simulink model "quadrotorsim"  (Simulink 9.2)
settings: Solver=ode45  StartTime=0.0  StopTime=200  FixedStep=1  RelTol=1e-3  EnableMultiTasking=on
undefined symbols (not defined in the file): delta_th_lim, delta_w_lim, Fmat, Hmat, KfupdatePeriodInCycle, max_bias, Q, q0, qest0, R, Tcapt, TkfProp, Tqint
libraries: simulink x2
settings Model: Creator=samirbo  LastModifiedBy=william
settings OptimizationCC: ExpressionDepthLimit=2147483647  InitFltsAndDblsToZero=on
settings DebuggingCC: SaveWithParameterizedLinksMsg=none  SignalResolutionControl=TryResolveAllWithWarning  SolverPrmCheckMsg=warning  MultiTaskDSMMsg=warning  MultiTaskCondExecSysMsg=none
settings GRTTargetCC: TargetFcnLib=ansi_tfl_tmw.mat

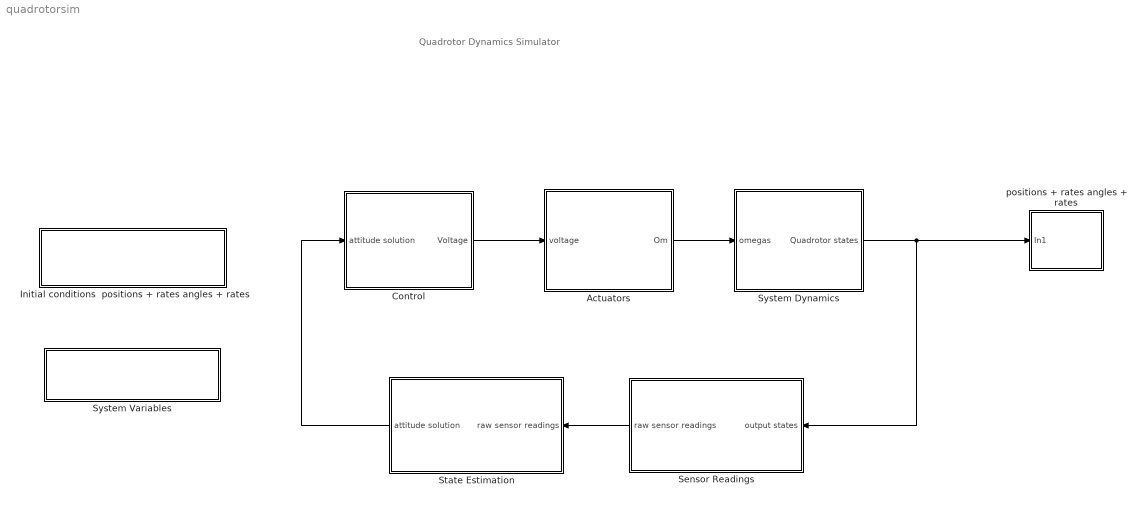
== system quadrotorsim ==
  note: Quadrotor Dynamics Simulator
  Actuators : Subsystem
      mask Display: image(imread('Brushless-motor.jpg'))
  Control : Subsystem
      mask Display: image(imread('control.bmp'))
  Initial conditions  positions + rates angles + rates : Subsystem  mask{x0=5, y0=5, z0=5, x0dot=1, y0dot=1, z0dot=1, phi0=0, theta0=0, psi0=0, phi0dot=0, theta0dot=0, psi0dot=0}
      mask prompts: x0 "Initial X position, in meters"; y0 "Initial Y position, in meters"; z0 "Initial Z position, in meters"; x0dot "Initial Velocity in X direction, m/sec"; y0dot "Initial Velocity in Y direction, m/sec"; z0dot "Initial Velocity in Z direction, m/sec"; phi0 "Initial Roll angle, deg"; theta0 "Initial Pitch angle, deg"; psi0 "Initial Yaw angle, deg"; phi0dot "Initial Roll rate, deg/sec"; theta0dot "Initial Pitch rate, deg/sec"; psi0dot "Initial Yaw rate, deg/sec"
      mask Display: disp('Enter initial conditions here')
  Sensor Readings : Subsystem
      mask Display: image(imread('imu.jpg'))
  State Estimation : Subsystem
      mask Display: image(imread('filter.png'))
  System Dynamics : Subsystem
      mask Display: image(imread('Quadrotor.png'))
  System Variables : Subsystem  mask{m=5, Ixx=0.03, Iyy=0.03, Izz=0.03, b=1, d=0.6, Jr=0.01, l=0.5}
      mask prompts: m "Quadrotor Mass, in kg"; Ixx "Quadrotor Moment of Inertia along x axis, in kg.m^2"; Iyy "Quadrotor Moment of Inertia along y axis, in kg.m^2"; Izz "Quadrotor Moment of Inertia along z axix, kg.m^2"; b "Thrust Factor"; d "Drag factor"; Jr "Rotor Inertia, in kg.m^2"; l "Length from the rotor to the centre of mass, in m"
      mask Display: disp('input system variables')
  positions + rates angles + rates : Subsystem
      mask Display: disp('system states')
  wires:
  Actuators/1(Om) -> System Dynamics/1(omegas)
  System Dynamics/1(Quadrotor states) -> Sensor Readings/1(output states), positions + rates angles + rates/1(In1)
  Sensor Readings/1(raw sensor readings) -> State Estimation/1(raw sensor readings)
  Control/1(Voltage) -> Actuators/1(voltage)
  State Estimation/1(attitude solution) -> Control/1(attitude solution)

== system quadrotorsim/Actuators ==
  voltage : Inport
  Bus Creator : BusCreator  Inputs=4
  Bus Selector : BusSelector  OutputSignals=d
  "Motor Dynamics - Front Motor " : Subsystem  mask{Jm=0.001, Jp=0.01, R=0.1, Ke=23}
      mask prompts: Jm "Total Moment of Inertia of the motor in the spin axis, N m s^2"; Jp "Total Moment of Inertia of the propeller in the spin axis, N m s^2"; R "Internal resistance of the motor, Ohm"; Ke "Motor constant, V/rad/sec"
  Motor Dynamics - Left Motor : Subsystem  mask{Jm=0.001, Jp=0.01, R=0.1, Ke=23}
      mask prompts: Jm "Total Moment of Inertia of the motor in the spin axis, N m s^2"; Jp "Total Moment of Inertia of the propeller in the spin axis, N m s^2"; R "Internal resistance of the motor, Ohm"; Ke "Motor constant, V/rad/sec"
  Motor Dynamics - Rear Motor : Subsystem  mask{Jm=0.001, Jp=0.01, R=0.1, Ke=23}
      mask prompts: Jm "Total Moment of Inertia of the motor in the spin axis, N m s^2"; Jp "Total Moment of Inertia of the propeller in the spin axis, N m s^2"; R "Internal resistance of the motor, Ohm"; Ke "Motor constant, V/rad/sec"
  Motor Dynamics - Right Motor : Subsystem  mask{Jm=0.001, Jp=0.01, R=0.1, Ke=23}
      mask prompts: Jm "Total Moment of Inertia of the motor in the spin axis, N m s^2"; Jp "Total Moment of Inertia of the propeller in the spin axis, N m s^2"; R "Internal resistance of the motor, Ohm"; Ke "Motor constant, V/rad/sec"
  Om : Outport
  wires:
  [SystemVariables] -> Bus Selector/1
  Bus Selector/1 -> Motor Dynamics - Right Motor/2(drag coefficient), Motor Dynamics - Rear Motor/2(drag coefficient), Motor Dynamics - Left Motor/2(drag coefficient), "Motor Dynamics - Front Motor "/2(drag coefficient)  "<d>"
  voltage/1 -> "Motor Dynamics - Front Motor "/1(voltage), Motor Dynamics - Right Motor/1(voltage), Motor Dynamics - Rear Motor/1(voltage), Motor Dynamics - Left Motor/1(voltage)
  "Motor Dynamics - Front Motor "/1(RPS) -> Bus Creator/1  "Om_1"
  Motor Dynamics - Right Motor/1(RPS) -> Bus Creator/2  "Om_2"
  Motor Dynamics - Rear Motor/1(RPS) -> Bus Creator/3  "Om_3"
  Motor Dynamics - Left Motor/1(RPS) -> Bus Creator/4  "Om_4"
  Bus Creator/1 -> Om/1

== system quadrotorsim/Control ==
  attitude solution : Inport
  Bus Selector : BusSelector  OutputSignals=west
  Voltage conversion : Gain
  attitude controller : Subsystem
  steering commands : Subsystem
  Voltage : Outport
  wires:
  steering commands/1(wstr) -> attitude controller/1(wstr)
  attitude solution/1 -> Bus Selector/1
  Bus Selector/1 -> attitude controller/2(west)  "<west>"
  attitude controller/1(trq) -> Voltage conversion/1
  Voltage conversion/1 -> Voltage/1

== system quadrotorsim/Initial conditions  positions + rates angles + rates ==
  note: positions and linear velocities
  note: angles and angular velocities
  note: yaw
  note: pitch
  note: roll
  Bus Creator : BusCreator  Inputs=12
  phi [rad] : Constant  Value=phi0
  phidot [rad/s] : Constant  Value=phi0dot
  psi [rad] : Constant  Value=psi0
  psidot [rad/s] : Constant  Value=psi0dot
  theta [rad] : Constant  Value=theta0
  thetadot [rad/s] : Constant  Value=theta0dot
  x [m] : Constant  Value=x0
  xdot [m/s] : Constant  Value=x0dot
  y [m] : Constant  Value=y0
  ydot [m/s] : Constant  Value=y0dot
  z [m] : Constant  Value=z0
  zdot [m/s] : Constant  Value=z0dot
  tag scope: InitialConditions=global
  wires:
  x [m]/1 -> Bus Creator/1  "x0"
  xdot [m/s]/1 -> Bus Creator/2  "x0dot"
  y [m]/1 -> Bus Creator/3  "y0"
  ydot [m/s]/1 -> Bus Creator/4  "y0dot"
  z [m]/1 -> Bus Creator/5  "z0"
  zdot [m/s]/1 -> Bus Creator/6  "z0dot"
  phi [rad]/1 -> Bus Creator/7  "phi0"
  phidot [rad/s]/1 -> Bus Creator/8  "phi0dot"
  theta [rad]/1 -> Bus Creator/9  "theta0"
  thetadot [rad/s]/1 -> Bus Creator/10  "theta0dot"
  psi [rad]/1 -> Bus Creator/11  "psi0"
  psidot [rad/s]/1 -> Bus Creator/12  "psi0dot"
  Bus Creator/1 -> [InitialConditions]

== system quadrotorsim/Sensor Readings ==
  note: Senor output values in 13 bits
  output states : Inport
  Altitude Sensor : Subsystem
  Rate Sensor Unit : Subsystem
  Terminator : Terminator
  raw sensor readings : Outport
  wires:
  output states/1 -> Rate Sensor Unit/1(In1), Altitude Sensor/1(In1)
  Rate Sensor Unit/1(Out1) -> raw sensor readings/1  "RSoutput"
  Altitude Sensor/1(Out1) -> Terminator/1  "sonaroutput"

== system quadrotorsim/State Estimation ==
  raw sensor readings : Inport
  ADC conversion : Subsystem
  Bus Creator : BusCreator  Inputs=2
  attitude estimator : Subsystem
  kinematics: dq/dt = 1/2 Wq : Subsystem
  attitude solution : Outport
  wires:
  kinematics: dq/dt = 1/2 Wq/1(q) -> attitude estimator/1(q)
  attitude estimator/1(qest) -> Bus Creator/1  "qest"
  attitude estimator/2(west) -> Bus Creator/2  "west"
  Bus Creator/1 -> attitude solution/1  "attsol"
  raw sensor readings/1 -> ADC conversion/1(In1)
  ADC conversion/1(w) -> kinematics: dq/dt = 1/2 Wq/1(w), attitude estimator/2(w)

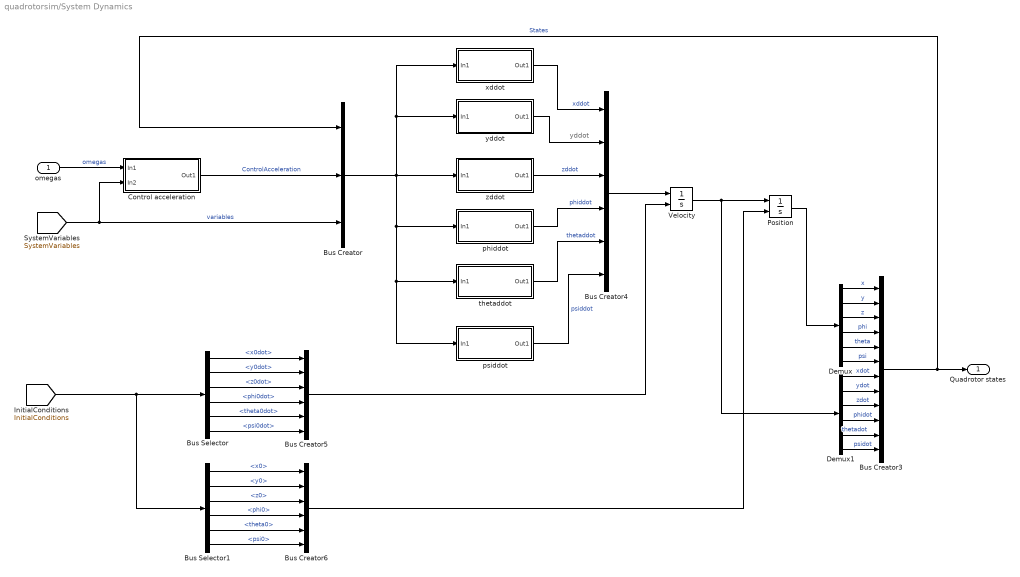
== system quadrotorsim/System Dynamics ==
  note: yddot
  omegas : Inport
  Bus Creator : BusCreator  Inputs=3
  Bus Creator3 : BusCreator  Inputs=12
  Bus Creator4 : BusCreator  Inputs=6
  Bus Creator5 : BusCreator  Inputs=6
  Bus Creator6 : BusCreator  Inputs=6
  Bus Selector : BusSelector  OutputSignals=x0dot,y0dot,z0dot,phi0dot,theta0dot,psi0dot
  Bus Selector1 : BusSelector  OutputSignals=x0,y0,z0,phi0,theta0,psi0
  Control acceleration : Subsystem
  Demux : Demux  Outputs=6
  Demux1 : Demux  Outputs=6
  Position : Integrator  InitialConditionSource=external
  Velocity : Integrator  InitialConditionSource=external
  phiddot : Subsystem
  psiddot : Subsystem
  thetaddot : Subsystem
  xddot : Subsystem
  yddot : Subsystem
  zddot : Subsystem
  Quadrotor states : Outport
  wires:
  [SystemVariables] -> Bus Creator/3, Control acceleration/2(In2)  "variables"
  Control acceleration/1(Out1) -> Bus Creator/2  "ControlAcceleration"
  omegas/1 -> Control acceleration/1(In1)  "omegas"
  Bus Creator/1 -> xddot/1(In1), yddot/1(In1), zddot/1(In1), phiddot/1(In1), thetaddot/1(In1), psiddot/1(In1)
  xddot/1(Out1) -> Bus Creator4/1  "xddot"
  yddot/1(Out1) -> Bus Creator4/2
  zddot/1(Out1) -> Bus Creator4/3  "zddot"
  phiddot/1(Out1) -> Bus Creator4/4  "phiddot"
  thetaddot/1(Out1) -> Bus Creator4/5  "thetaddot"
  psiddot/1(Out1) -> Bus Creator4/6  "psiddot"
  Position/1 -> Demux/1
  Bus Creator4/1 -> Velocity/1
  Velocity/1 -> Position/1, Demux1/1
  [InitialConditions] -> Bus Selector/1, Bus Selector1/1
  Bus Selector/1 -> Bus Creator5/1  "<x0dot>"
  Bus Selector/2 -> Bus Creator5/2  "<y0dot>"
  Bus Selector/3 -> Bus Creator5/3  "<z0dot>"
  Bus Selector/4 -> Bus Creator5/4  "<phi0dot>"
  Bus Selector/5 -> Bus Creator5/5  "<theta0dot>"
  Bus Selector/6 -> Bus Creator5/6  "<psi0dot>"
  Bus Creator5/1 -> Velocity/2
  Bus Selector1/1 -> Bus Creator6/1  "<x0>"
  Bus Selector1/2 -> Bus Creator6/2  "<y0>"
  Bus Selector1/3 -> Bus Creator6/3  "<z0>"
  Bus Selector1/4 -> Bus Creator6/4  "<phi0>"
  Bus Selector1/5 -> Bus Creator6/5  "<theta0>"
  Bus Selector1/6 -> Bus Creator6/6  "<psi0>"
  Bus Creator6/1 -> Position/2
  Demux/1 -> Bus Creator3/1  "x"
  Demux/2 -> Bus Creator3/2  "y"
  Demux/3 -> Bus Creator3/3  "z"
  Demux/4 -> Bus Creator3/4  "phi"
  Demux/5 -> Bus Creator3/5  "theta"
  Demux/6 -> Bus Creator3/6  "psi"
  Demux1/1 -> Bus Creator3/7  "xdot"
  Demux1/2 -> Bus Creator3/8  "ydot"
  Demux1/3 -> Bus Creator3/9  "zdot"
  Demux1/4 -> Bus Creator3/10  "phidot"
  Demux1/5 -> Bus Creator3/11  "thetadot"
  Demux1/6 -> Bus Creator3/12  "psidot"
  Bus Creator3/1 -> Quadrotor states/1, Bus Creator/1  "States"

== system quadrotorsim/System Variables ==
  Bus Creator : BusCreator  Inputs=8
  Drag Factor : Constant  Value=d
  InertiaX : Constant  Value=Ixx
  InertiaY : Constant  Value=Iyy
  InertiaZ : Constant  Value=Izz
  Length : Constant  Value=l
  Quadrotor Mass : Constant  Value=m
  Rotor Inertia : Constant  Value=Jr
  Thrust Factor : Constant  Value=b
  tag scope: SystemVariables=global
  wires:
  Bus Creator/1 -> [SystemVariables]
  Quadrotor Mass/1 -> Bus Creator/1  "m"
  InertiaX/1 -> Bus Creator/2  "Ixx"
  InertiaY/1 -> Bus Creator/3  "Iyy"
  InertiaZ/1 -> Bus Creator/4  "Izz"
  Thrust Factor/1 -> Bus Creator/5  "b"
  Drag Factor/1 -> Bus Creator/6  "d"
  Rotor Inertia/1 -> Bus Creator/7  "Jr"
  Length/1 -> Bus Creator/8  "l"

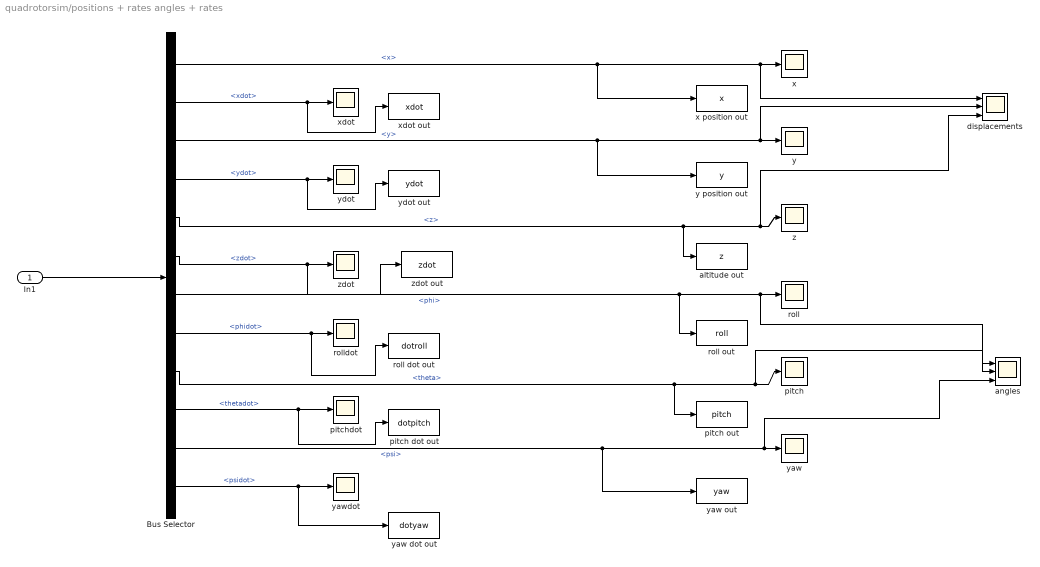
== system quadrotorsim/positions + rates angles + rates ==
  In1 : Inport
  Bus Selector : BusSelector  OutputSignals=x,xdot,y,ydot,z,zdot,phi,phidot,theta,thetadot,psi,psidot
  altitude out : ToWorkspace  VariableName=z  SampleTime=-1
  angles : Scope  NumInputPorts=3
  displacements : Scope  NumInputPorts=3
  pitch : Scope
  pitch dot out : ToWorkspace  VariableName=dotpitch  SampleTime=-1
  pitch out : ToWorkspace  VariableName=pitch  SampleTime=-1
  pitchdot : Scope
  roll : Scope
  roll dot out : ToWorkspace  VariableName=dotroll  SampleTime=-1
  roll out : ToWorkspace  VariableName=roll  SampleTime=-1
  rolldot : Scope
  x : Scope
  x position out : ToWorkspace  VariableName=x  SampleTime=-1
  xdot : Scope
  xdot out : ToWorkspace  VariableName=xdot  SampleTime=-1
  y : Scope
  y position out : ToWorkspace  VariableName=y  SampleTime=-1
  yaw : Scope
  yaw dot out : ToWorkspace  VariableName=dotyaw  SampleTime=-1
  yaw out : ToWorkspace  VariableName=yaw  SampleTime=-1
  yawdot : Scope
  ydot : Scope
  ydot out : ToWorkspace  VariableName=ydot  SampleTime=-1
  z : Scope
  zdot : Scope
  zdot out : ToWorkspace  VariableName=zdot  SampleTime=-1
  wires:
  Bus Selector/2 -> xdot/1, xdot out/1  "<xdot>"
  Bus Selector/4 -> ydot/1, ydot out/1  "<ydot>"
  Bus Selector/1 -> x position out/1, x/1, displacements/1  "<x>"
  Bus Selector/3 -> y position out/1, y/1, displacements/2  "<y>"
  Bus Selector/12 -> yawdot/1, yaw dot out/1  "<psidot>"
  Bus Selector/11 -> yaw out/1, yaw/1, angles/3  "<psi>"
  In1/1 -> Bus Selector/1
  Bus Selector/10 -> pitchdot/1, pitch dot out/1  "<thetadot>"
  Bus Selector/5 -> altitude out/1, z/1, displacements/3  "<z>"
  Bus Selector/6 -> zdot/1, zdot out/1  "<zdot>"
  Bus Selector/7 -> roll out/1, roll/1, angles/1  "<phi>"
  Bus Selector/8 -> rolldot/1, roll dot out/1  "<phidot>"
  Bus Selector/9 -> pitch out/1, pitch/1, angles/2  "<theta>"

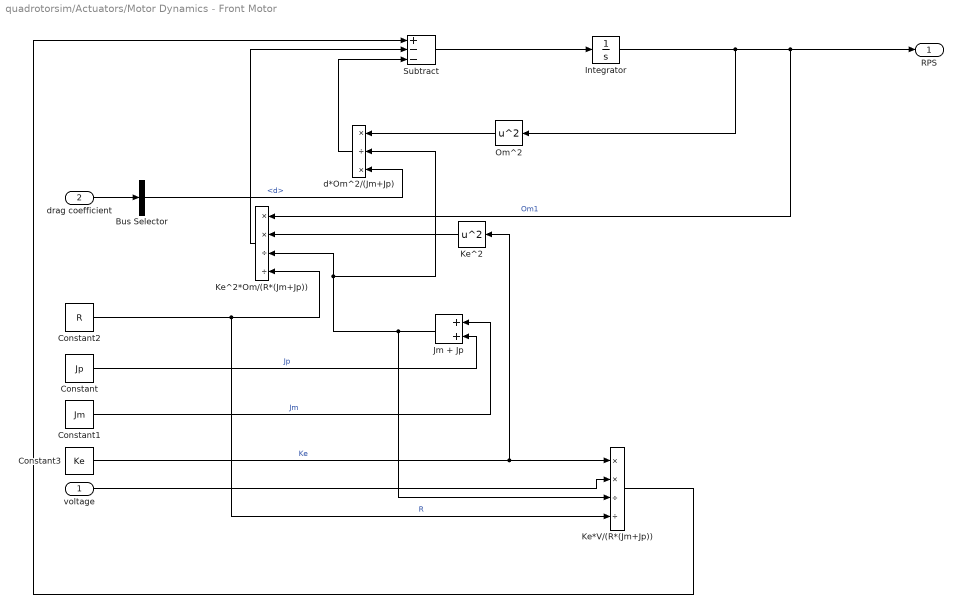
== system quadrotorsim/Actuators/Motor Dynamics - Front Motor  ==
  voltage : Inport
  drag coefficient : Inport  Port=2
  Bus Selector : BusSelector  OutputSignals=d
  Constant : Constant  Value=Jp
  Constant1 : Constant  Value=Jm
  Constant2 : Constant  Value=R
  Constant3 : Constant  Value=Ke
  Integrator : Integrator
  Jm + Jp : Sum
  Ke*V/(R*(Jm+Jp)) : Product  Inputs=**//  RndMeth=Zero
  Ke^2 : Math  Operator=square  SaturateOnIntegerOverflow=on
  Ke^2*Om/(R*(Jm+Jp)) : Product  Inputs=**//  RndMeth=Zero
  Om^2 : Math  Operator=square  SaturateOnIntegerOverflow=on
  Subtract : Sum  Inputs=+--
  d*Om^2/(Jm+Jp) : Product  Inputs=*/*  RndMeth=Zero
  RPS : Outport
  wires:
  Integrator/1 -> RPS/1, Ke^2*Om/(R*(Jm+Jp))/1, Om^2/1  "Om1"
  Constant/1 -> Jm + Jp/2  "Jp"
  Constant1/1 -> Jm + Jp/1  "Jm"
  Constant2/1 -> Ke^2*Om/(R*(Jm+Jp))/4, Ke*V/(R*(Jm+Jp))/4  "R"
  Constant3/1 -> Ke^2/1, Ke*V/(R*(Jm+Jp))/1  "Ke"
  Ke^2/1 -> Ke^2*Om/(R*(Jm+Jp))/2
  Jm + Jp/1 -> Ke^2*Om/(R*(Jm+Jp))/3, d*Om^2/(Jm+Jp)/2, Ke*V/(R*(Jm+Jp))/3
  Om^2/1 -> d*Om^2/(Jm+Jp)/1
  drag coefficient/1 -> Bus Selector/1
  Bus Selector/1 -> d*Om^2/(Jm+Jp)/3  "<d>"
  voltage/1 -> Ke*V/(R*(Jm+Jp))/2
  Ke*V/(R*(Jm+Jp))/1 -> Subtract/1
  Ke^2*Om/(R*(Jm+Jp))/1 -> Subtract/2
  d*Om^2/(Jm+Jp)/1 -> Subtract/3
  Subtract/1 -> Integrator/1

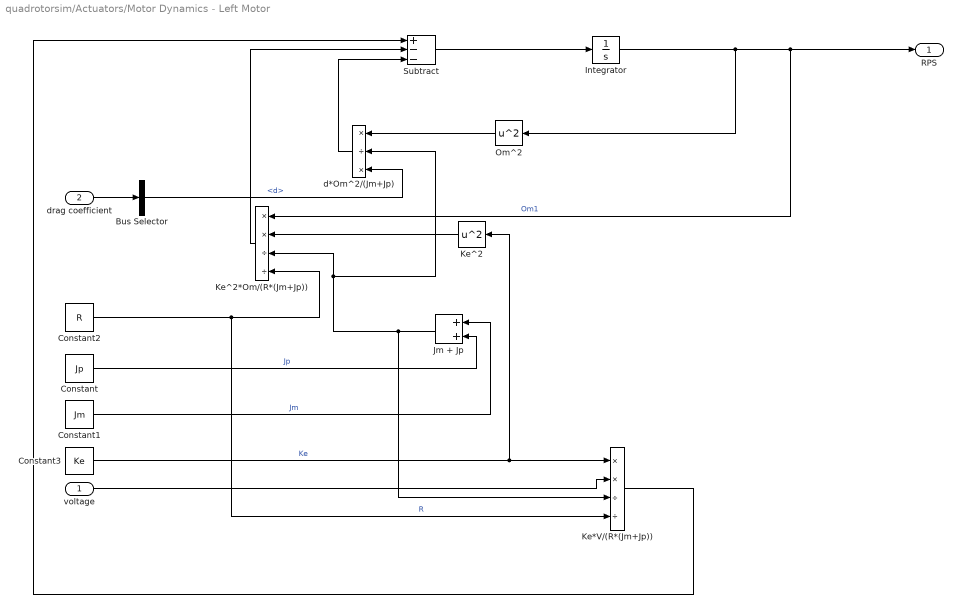
== system quadrotorsim/Actuators/Motor Dynamics - Left Motor ==
  voltage : Inport
  drag coefficient : Inport  Port=2
  Bus Selector : BusSelector  OutputSignals=d
  Constant : Constant  Value=Jp
  Constant1 : Constant  Value=Jm
  Constant2 : Constant  Value=R
  Constant3 : Constant  Value=Ke
  Integrator : Integrator
  Jm + Jp : Sum
  Ke*V/(R*(Jm+Jp)) : Product  Inputs=**//  RndMeth=Zero
  Ke^2 : Math  Operator=square  SaturateOnIntegerOverflow=on
  Ke^2*Om/(R*(Jm+Jp)) : Product  Inputs=**//  RndMeth=Zero
  Om^2 : Math  Operator=square  SaturateOnIntegerOverflow=on
  Subtract : Sum  Inputs=+--
  d*Om^2/(Jm+Jp) : Product  Inputs=*/*  RndMeth=Zero
  RPS : Outport
  wires:
  Subtract/1 -> Integrator/1
  d*Om^2/(Jm+Jp)/1 -> Subtract/3
  Ke^2*Om/(R*(Jm+Jp))/1 -> Subtract/2
  Ke*V/(R*(Jm+Jp))/1 -> Subtract/1
  voltage/1 -> Ke*V/(R*(Jm+Jp))/2
  Bus Selector/1 -> d*Om^2/(Jm+Jp)/3  "<d>"
  drag coefficient/1 -> Bus Selector/1
  Om^2/1 -> d*Om^2/(Jm+Jp)/1
  Jm + Jp/1 -> Ke*V/(R*(Jm+Jp))/3, d*Om^2/(Jm+Jp)/2, Ke^2*Om/(R*(Jm+Jp))/3
  Ke^2/1 -> Ke^2*Om/(R*(Jm+Jp))/2
  Constant3/1 -> Ke*V/(R*(Jm+Jp))/1, Ke^2/1  "Ke"
  Constant2/1 -> Ke*V/(R*(Jm+Jp))/4, Ke^2*Om/(R*(Jm+Jp))/4  "R"
  Constant1/1 -> Jm + Jp/1  "Jm"
  Constant/1 -> Jm + Jp/2  "Jp"
  Integrator/1 -> Om^2/1, Ke^2*Om/(R*(Jm+Jp))/1, RPS/1  "Om1"

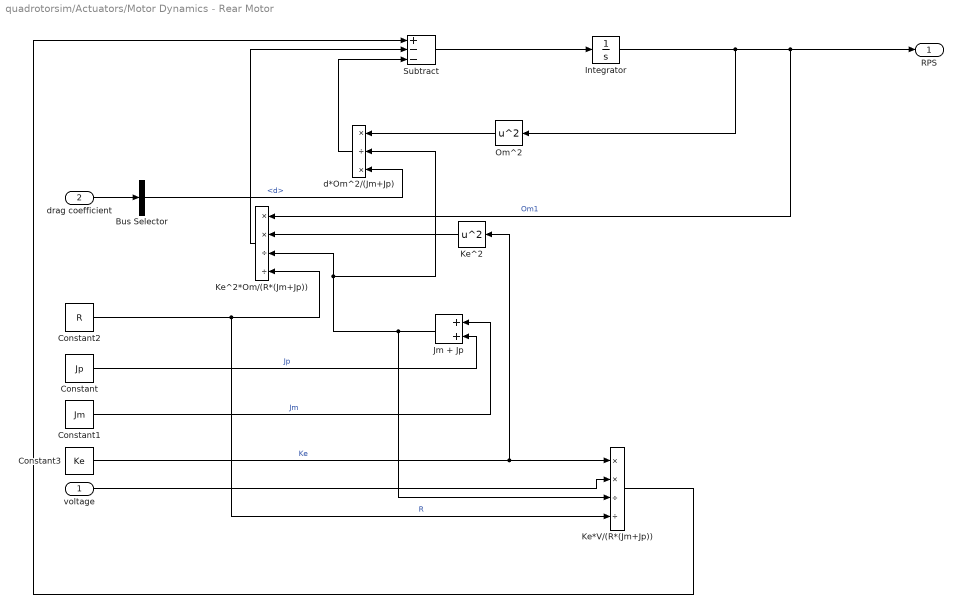
== system quadrotorsim/Actuators/Motor Dynamics - Rear Motor ==
  voltage : Inport
  drag coefficient : Inport  Port=2
  Bus Selector : BusSelector  OutputSignals=d
  Constant : Constant  Value=Jp
  Constant1 : Constant  Value=Jm
  Constant2 : Constant  Value=R
  Constant3 : Constant  Value=Ke
  Integrator : Integrator
  Jm + Jp : Sum
  Ke*V/(R*(Jm+Jp)) : Product  Inputs=**//  RndMeth=Zero
  Ke^2 : Math  Operator=square  SaturateOnIntegerOverflow=on
  Ke^2*Om/(R*(Jm+Jp)) : Product  Inputs=**//  RndMeth=Zero
  Om^2 : Math  Operator=square  SaturateOnIntegerOverflow=on
  Subtract : Sum  Inputs=+--
  d*Om^2/(Jm+Jp) : Product  Inputs=*/*  RndMeth=Zero
  RPS : Outport
  wires:
  Integrator/1 -> RPS/1, Ke^2*Om/(R*(Jm+Jp))/1, Om^2/1  "Om1"
  Constant/1 -> Jm + Jp/2  "Jp"
  Constant1/1 -> Jm + Jp/1  "Jm"
  Constant2/1 -> Ke^2*Om/(R*(Jm+Jp))/4, Ke*V/(R*(Jm+Jp))/4  "R"
  Constant3/1 -> Ke^2/1, Ke*V/(R*(Jm+Jp))/1  "Ke"
  Ke^2/1 -> Ke^2*Om/(R*(Jm+Jp))/2
  Jm + Jp/1 -> Ke^2*Om/(R*(Jm+Jp))/3, d*Om^2/(Jm+Jp)/2, Ke*V/(R*(Jm+Jp))/3
  Om^2/1 -> d*Om^2/(Jm+Jp)/1
  drag coefficient/1 -> Bus Selector/1
  Bus Selector/1 -> d*Om^2/(Jm+Jp)/3  "<d>"
  voltage/1 -> Ke*V/(R*(Jm+Jp))/2
  Ke*V/(R*(Jm+Jp))/1 -> Subtract/1
  Ke^2*Om/(R*(Jm+Jp))/1 -> Subtract/2
  d*Om^2/(Jm+Jp)/1 -> Subtract/3
  Subtract/1 -> Integrator/1

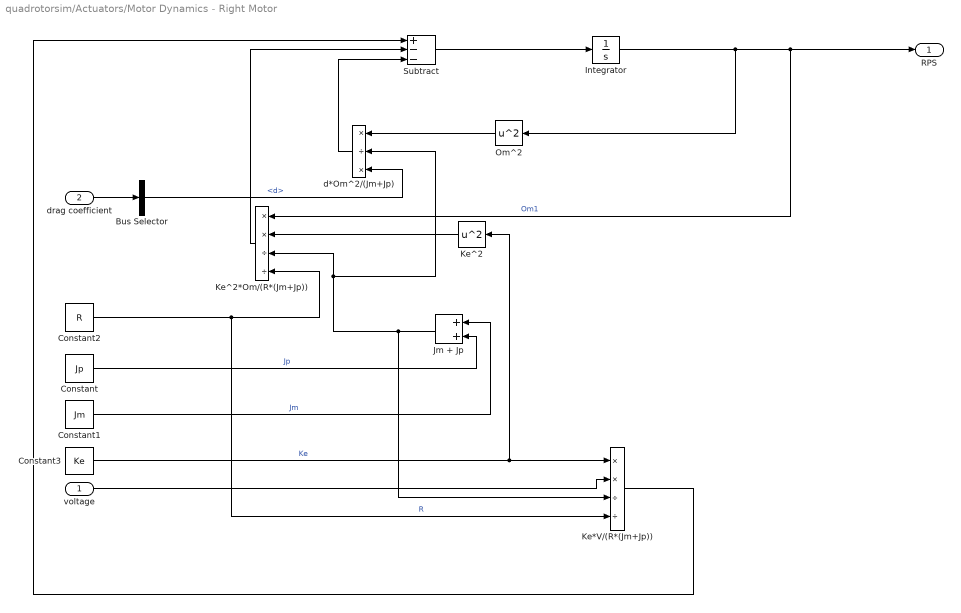
== system quadrotorsim/Actuators/Motor Dynamics - Right Motor ==
  voltage : Inport
  drag coefficient : Inport  Port=2
  Bus Selector : BusSelector  OutputSignals=d
  Constant : Constant  Value=Jp
  Constant1 : Constant  Value=Jm
  Constant2 : Constant  Value=R
  Constant3 : Constant  Value=Ke
  Integrator : Integrator
  Jm + Jp : Sum
  Ke*V/(R*(Jm+Jp)) : Product  Inputs=**//  RndMeth=Zero
  Ke^2 : Math  Operator=square  SaturateOnIntegerOverflow=on
  Ke^2*Om/(R*(Jm+Jp)) : Product  Inputs=**//  RndMeth=Zero
  Om^2 : Math  Operator=square  SaturateOnIntegerOverflow=on
  Subtract : Sum  Inputs=+--
  d*Om^2/(Jm+Jp) : Product  Inputs=*/*  RndMeth=Zero
  RPS : Outport
  wires:
  Subtract/1 -> Integrator/1
  d*Om^2/(Jm+Jp)/1 -> Subtract/3
  Ke^2*Om/(R*(Jm+Jp))/1 -> Subtract/2
  Ke*V/(R*(Jm+Jp))/1 -> Subtract/1
  voltage/1 -> Ke*V/(R*(Jm+Jp))/2
  Bus Selector/1 -> d*Om^2/(Jm+Jp)/3  "<d>"
  drag coefficient/1 -> Bus Selector/1
  Om^2/1 -> d*Om^2/(Jm+Jp)/1
  Jm + Jp/1 -> Ke*V/(R*(Jm+Jp))/3, d*Om^2/(Jm+Jp)/2, Ke^2*Om/(R*(Jm+Jp))/3
  Ke^2/1 -> Ke^2*Om/(R*(Jm+Jp))/2
  Constant3/1 -> Ke*V/(R*(Jm+Jp))/1, Ke^2/1  "Ke"
  Constant2/1 -> Ke*V/(R*(Jm+Jp))/4, Ke^2*Om/(R*(Jm+Jp))/4  "R"
  Constant1/1 -> Jm + Jp/1  "Jm"
  Constant/1 -> Jm + Jp/2  "Jp"
  Integrator/1 -> Om^2/1, Ke^2*Om/(R*(Jm+Jp))/1, RPS/1  "Om1"

== system quadrotorsim/Control/attitude controller ==
  wstr : Inport
  west : Inport  Port=2
  Add : Sum  Inputs=+-
  Gain : Gain  Gain=0
  trq : Outport
  wires:
  wstr/1 -> Add/1
  west/1 -> Add/2
  Add/1 -> Gain/1
  Gain/1 -> trq/1

== system quadrotorsim/Control/steering commands ==
  Constant4 : Constant  Value=[0,0,0]
  wstr : Outport
  wires:
  Constant4/1 -> wstr/1

== system quadrotorsim/Sensor Readings/Altitude Sensor ==
  In1 : Inport
  Sonar : Subsystem
  Out1 : Outport
  wires:
  Sonar/1(Altitude) -> Out1/1  "Alt.Sonar"
  In1/1 -> Sonar/1(In1)

== system quadrotorsim/Sensor Readings/Rate Sensor Unit ==
  In1 : Inport
  Bus Creator2 : BusCreator  Inputs=3
  Demux2 : Demux  Outputs=3
  Gyro : Subsystem
  Out1 : Outport
  wires:
  In1/1 -> Gyro/1(In1)
  Gyro/1(rates) -> Demux2/1
  Demux2/1 -> Bus Creator2/1  "RollRate.Gyro"
  Demux2/2 -> Bus Creator2/2  "PitchRate.Gyro"
  Demux2/3 -> Bus Creator2/3  "YawRate.Gyro"
  Bus Creator2/1 -> Out1/1  "GyroReading"

== system quadrotorsim/State Estimation/ADC conversion ==
  note: Conversion of bits to the engineering units (rad/sec)
  In1 : Inport
  Conversion of bits to the engineering units (rad/sec) : Gain  Gain=2000*pi/(8161*180)  OutDataTypeStr=double
  Demux : Demux  Outputs=3
  Gain2 : Gain  Gain=2000*pi/(8161*180)  OutDataTypeStr=double
  Gain3 : Gain  Gain=2000*pi/(8161*180)  OutDataTypeStr=double
  Mux : Mux  Inputs=3
  w : Outport
  wires:
  In1/1 -> Demux/1
  Demux/1 -> Conversion of bits to the engineering units (rad/sec)/1
  Demux/2 -> Gain2/1
  Demux/3 -> Gain3/1
  Conversion of bits to the engineering units (rad/sec)/1 -> Mux/1  "p"
  Gain2/1 -> Mux/2  "q"
  Gain3/1 -> Mux/3  "r"
  Mux/1 -> w/1  "w"

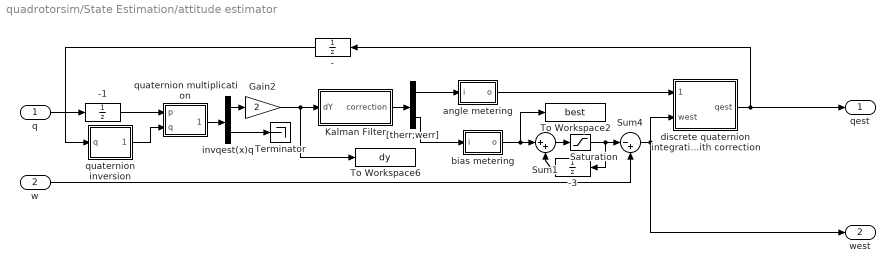
== system quadrotorsim/State Estimation/attitude estimator ==
  q : Inport
  w : Inport  Port=2
  - : UnitDelay  SampleTime=-1
  -1 : UnitDelay  SampleTime=-1
  -3 : UnitDelay  InitialCondition=[0;0;0]  SampleTime=-1
  Gain2 : Gain  Gain=2
  Kalman Filter : Subsystem
  Saturation : Saturate  UpperLimit=max_bias  LowerLimit=-max_bias
  Sum1 : Sum  Inputs=|++  SaturateOnIntegerOverflow=on  InputSameDT=on  OutDataTypeStr=Inherit: Same as first input
  Sum4 : Sum  Inputs=|-+  SaturateOnIntegerOverflow=on  InputSameDT=on  OutDataTypeStr=Inherit: Same as first input
  Terminator : Terminator
  To Workspace2 : ToWorkspace  VariableName=best  SampleTime=Tcapt
  To Workspace6 : ToWorkspace  VariableName=dy  SampleTime=Tcapt
  "[therr;werr]" : Demux  Outputs=[3 3]
  angle metering : Subsystem
  bias metering : Subsystem
  discrete quaternion integration with correction : Subsystem
  invqest(x)q : Demux  Outputs=[3 1]
  quaternion inversion : Subsystem
  quaternion multiplication : Subsystem
  qest : Outport
  west : Outport  Port=2
  wires:
  q/1 -> -1/1
  invqest(x)q/2 -> Terminator/1
  invqest(x)q/1 -> Gain2/1
  quaternion multiplication/1(p(x)q) -> invqest(x)q/1
  w/1 -> Sum4/2
  Sum4/1 -> discrete quaternion integration with correction/2(west), west/1
  -/1 -> quaternion inversion/1(q)
  Kalman Filter/1(correction) -> "[therr;werr]"/1
  "[therr;werr]"/1 -> angle metering/1(i)
  "[therr;werr]"/2 -> bias metering/1(i)
  Gain2/1 -> Kalman Filter/1(dY), To Workspace6/1
  bias metering/1(o) -> To Workspace2/1, Sum1/1
  angle metering/1(o) -> discrete quaternion integration with correction/1(correction)
  discrete quaternion integration with correction/1(qest) -> -/1, qest/1
  Sum1/1 -> Saturation/1
  -3/1 -> Sum1/2
  Saturation/1 -> -3/1, Sum4/1
  -1/1 -> quaternion multiplication/1(p)
  quaternion inversion/1(invq) -> quaternion multiplication/2(q)

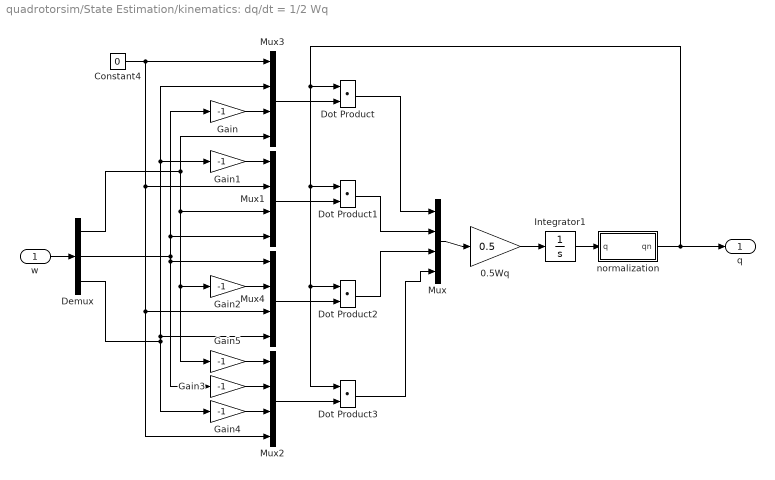
== system quadrotorsim/State Estimation/kinematics: dq/dt = 1/2 Wq ==
  w : Inport  OutDataTypeStr=double
  0.5Wq : Gain  Gain=0.5
  Constant4 : Constant  Value=0
  Demux : Demux  Outputs=3
  Dot Product{,1..3} (4 alike) : DotProduct  InputSameDT=on  OutDataTypeStr=Inherit: Inherit via internal rule
  Gain{,1..5} (6 alike) : Gain  Gain=-1
  Integrator1 : Integrator  InitialCondition=q0
  Mux{,1..4} (5 alike) : Mux
  normalization : Subsystem
  q : Outport
  wires:
  Gain2/1 -> Mux4/2
  Gain/1 -> Mux3/3
  Constant4/1 -> Mux3/1, Mux1/2, Mux2/4, Mux4/3
  Gain1/1 -> Mux1/1
  Gain5/1 -> Mux2/1
  Gain3/1 -> Mux2/2
  Gain4/1 -> Mux2/3
  Demux/1 -> Mux3/4, Mux1/3, Gain5/1, Gain2/1
  Demux/2 -> Gain/1, Mux1/4, Gain3/1, Mux4/1
  Demux/3 -> Gain4/1, Gain1/1, Mux3/2, Mux4/4
  Mux3/1 -> Dot Product/2
  Mux1/1 -> Dot Product1/2
  Mux4/1 -> Dot Product2/2
  Mux2/1 -> Dot Product3/2
  Dot Product/1 -> Mux/1
  Dot Product1/1 -> Mux/2
  Dot Product2/1 -> Mux/3
  Dot Product3/1 -> Mux/4
  Mux/1 -> 0.5Wq/1
  0.5Wq/1 -> Integrator1/1
  Integrator1/1 -> normalization/1(q)
  normalization/1(qn) -> q/1, Dot Product3/1, Dot Product2/1, Dot Product1/1, Dot Product/1
  w/1 -> Demux/1

== system quadrotorsim/System Dynamics/Control acceleration ==
  In1 : Inport
  In2 : Inport  Port=2
  Bus Creator : BusCreator  Inputs=5
  Bus Selector : BusSelector  OutputSignals=Om_1,Om_2,Om_3,Om_4
  Bus Selector1 : BusSelector  OutputSignals=b,d
  Mux : Mux  Inputs=6
  Om : Fcn  Expr=(u(2)+u(4)-u(1)-u(3))
  U1 : Fcn  Expr=u(5)*(u(1)^2+u(2)^2+u(3)^2+u(4)^2)
  U2 : Fcn  Expr=u(5)*(u(4)^2-u(2)^2)
  U3 : Fcn  Expr=u(5)*(u(3)^2-u(1)^2)
  U4 : Fcn  Expr=u(6)*(u(2)^2+u(4)^2-u(1)^2-u(3)^2)
  Out1 : Outport
  wires:
  In1/1 -> Bus Selector/1
  In2/1 -> Bus Selector1/1
  Bus Selector/1 -> Mux/1  "<Om_1>"
  Bus Selector/2 -> Mux/2  "<Om_2>"
  Bus Selector/3 -> Mux/3  "<Om_3>"
  Bus Selector/4 -> Mux/4  "<Om_4>"
  Bus Selector1/1 -> Mux/5  "<b>"
  Bus Selector1/2 -> Mux/6  "<d>"
  Mux/1 -> U1/1, U2/1, U3/1, U4/1, Om/1
  U1/1 -> Bus Creator/1  "U1"
  U2/1 -> Bus Creator/2  "U2"
  U3/1 -> Bus Creator/3  "U3"
  U4/1 -> Bus Creator/4  "U4"
  Om/1 -> Bus Creator/5  "Om"
  Bus Creator/1 -> Out1/1

== system quadrotorsim/System Dynamics/phiddot ==
  In1 : Inport
  Bus Selector : BusSelector  OutputSignals=States.thetadot,States.psidot,variables.Ixx,variables.Iyy,variables.Izz,variables.Jr,variables.l,ControlAcceleration.U2,ControlAcceleration.Om
  Fcn : Fcn  Expr=u(1)*u(2)*((u(4)-u(5))/u(3))-(u(6)*u(1)*u(9)/u(3))+(u(7)*u(8)/u(3))
  Mux : Mux  Inputs=9
  Out1 : Outport
  wires:
  Fcn/1 -> Out1/1
  Mux/1 -> Fcn/1
  In1/1 -> Bus Selector/1
  Bus Selector/3 -> Mux/3  "<Ixx>"
  Bus Selector/4 -> Mux/4  "<Iyy>"
  Bus Selector/5 -> Mux/5  "<Izz>"
  Bus Selector/6 -> Mux/6  "<Jr>"
  Bus Selector/7 -> Mux/7  "<l>"
  Bus Selector/8 -> Mux/8  "<U2>"
  Bus Selector/9 -> Mux/9  "<Om>"
  Bus Selector/2 -> Mux/2  "<psidot>"
  Bus Selector/1 -> Mux/1  "<thetadot>"

== system quadrotorsim/System Dynamics/psiddot ==
  In1 : Inport
  Bus Selector : BusSelector  OutputSignals=States.phidot,States.thetadot,variables.Ixx,variables.Iyy,variables.Izz,variables.l,ControlAcceleration.U4
  Fcn : Fcn  Expr=u(1)*u(2)*((u(3)-u(4))/u(5))+(u(6)*u(7)/u(5))
  Mux : Mux  Inputs=7
  Out1 : Outport
  wires:
  Fcn/1 -> Out1/1
  Mux/1 -> Fcn/1
  In1/1 -> Bus Selector/1
  Bus Selector/1 -> Mux/1  "<phidot>"
  Bus Selector/2 -> Mux/2  "<thetadot>"
  Bus Selector/3 -> Mux/3  "<Ixx>"
  Bus Selector/4 -> Mux/4  "<Iyy>"
  Bus Selector/5 -> Mux/5  "<Izz>"
  Bus Selector/6 -> Mux/6  "<l>"
  Bus Selector/7 -> Mux/7  "<U4>"

== system quadrotorsim/System Dynamics/thetaddot ==
  In1 : Inport
  Bus Selector : BusSelector  OutputSignals=States.phidot,States.psidot,variables.Iyy,variables.Izz,variables.Ixx,variables.Jr,variables.l,ControlAcceleration.U3,ControlAcceleration.Om
  Fcn : Fcn  Expr=u(1)*u(2)*((u(4)-u(5))/u(3))+(u(6)*u(1)*u(9)/u(3))+(u(7)*u(8)/u(3))
  Mux : Mux  Inputs=9
  Out1 : Outport
  wires:
  Bus Selector/1 -> Mux/1  "<phidot>"
  Bus Selector/2 -> Mux/2  "<psidot>"
  Bus Selector/9 -> Mux/9  "<Om>"
  Bus Selector/8 -> Mux/8  "<U3>"
  Bus Selector/7 -> Mux/7  "<l>"
  Bus Selector/6 -> Mux/6  "<Jr>"
  Bus Selector/3 -> Mux/4  "<Iyy>"
  In1/1 -> Bus Selector/1
  Mux/1 -> Fcn/1
  Fcn/1 -> Out1/1
  Bus Selector/4 -> Mux/3  "<Izz>"
  Bus Selector/5 -> Mux/5  "<Ixx>"

== system quadrotorsim/System Dynamics/xddot ==
  In1 : Inport
  Bus Selector : BusSelector  OutputSignals=States.phi,States.theta,States.psi,variables.m,ControlAcceleration.U1
  Fcn : Fcn  Expr=u(5)/u(4)*(cos(u(1))*sin(u(2))*cos(u(3))+sin(u(1))*sin(u(3)))
  Mux : Mux  Inputs=5
  Out1 : Outport
  wires:
  In1/1 -> Bus Selector/1
  Bus Selector/1 -> Mux/1  "<phi>"
  Bus Selector/2 -> Mux/2  "<theta>"
  Bus Selector/3 -> Mux/3  "<psi>"
  Bus Selector/4 -> Mux/4  "<m>"
  Bus Selector/5 -> Mux/5  "<U1>"
  Mux/1 -> Fcn/1
  Fcn/1 -> Out1/1

== system quadrotorsim/System Dynamics/yddot ==
  In1 : Inport
  Bus Selector : BusSelector  OutputSignals=States.phi,States.theta,States.psi,variables.m,ControlAcceleration.U1
  Fcn : Fcn  Expr=u(5)/u(4)*(cos(u(1))*sin(u(2))*sin(u(3))-sin(u(1))*cos(u(3)))
  Mux : Mux  Inputs=5
  Out1 : Outport
  wires:
  Fcn/1 -> Out1/1
  Mux/1 -> Fcn/1
  Bus Selector/5 -> Mux/5  "<U1>"
  Bus Selector/4 -> Mux/4  "<m>"
  Bus Selector/3 -> Mux/3  "<psi>"
  Bus Selector/2 -> Mux/2  "<theta>"
  Bus Selector/1 -> Mux/1  "<phi>"
  In1/1 -> Bus Selector/1

== system quadrotorsim/System Dynamics/zddot ==
  In1 : Inport
  Bus Selector : BusSelector  OutputSignals=States.phi,States.theta,variables.m,ControlAcceleration.U1
  Fcn : Fcn  Expr=u(4)/u(3)*(cos(u(1))*cos(u(2)))
  Mux : Mux
  Subtract : Sum  Inputs=+-
  gravitational acceleration : Constant  Value=9.81
  Out1 : Outport
  wires:
  In1/1 -> Bus Selector/1
  Bus Selector/1 -> Mux/1  "<phi>"
  Bus Selector/2 -> Mux/2  "<theta>"
  Mux/1 -> Fcn/1
  Bus Selector/3 -> Mux/3  "<m>"
  Bus Selector/4 -> Mux/4  "<U1>"
  Fcn/1 -> Subtract/1
  gravitational acceleration/1 -> Subtract/2
  Subtract/1 -> Out1/1

== system quadrotorsim/Sensor Readings/Altitude Sensor/Sonar ==
  In1 : Inport
  Add : Sum
  Band-Limited White Noise : simulink/Sources/Band-Limited White Noise  Cov=[0.1]  Ts=0.1  seed=[23341]
  Bus Selector : BusSelector  OutputSignals=z
  NoiseON/OFF : Gain  Gain=0
  Rate Transition : RateTransition  OutPortSampleTime=0.01
  y : Scope
  Altitude : Outport
  wires:
  In1/1 -> Bus Selector/1
  Bus Selector/1 -> Rate Transition/1  "<z>"
  NoiseON/OFF/1 -> Add/2
  Rate Transition/1 -> Add/1
  Band-Limited White Noise/1 -> NoiseON/OFF/1
  Add/1 -> Altitude/1

== system quadrotorsim/Sensor Readings/Rate Sensor Unit/Gyro ==
  note: Resolution of Gyro is assumed to be 2000 deg/sec
  In1 : Inport
  Add : Sum
  Band-Limited White Noise : simulink/Sources/Band-Limited White Noise  Cov=[0.1]  Ts=0.1  seed=[23341]
  Bus Creator : BusCreator  Inputs=3
  Bus Selector : BusSelector  OutputSignals=phidot,thetadot,psidot
  ConversiontoBits : Gain  Gain=(2^13-1)/2000
  Data Type Conversion : DataTypeConversion  OutDataTypeStr=uint16
  NoiseON/OFF : Gain
  RadtoDeg : Gain  Gain=180/pi
  Rate Transition : RateTransition  OutPortSampleTime=0.01
  Saturation : Saturate  UpperLimit=8191  LowerLimit=-8191
  rates : Outport
  wires:
  Bus Creator/1 -> Rate Transition/1
  Band-Limited White Noise/1 -> NoiseON/OFF/1
  Rate Transition/1 -> RadtoDeg/1
  RadtoDeg/1 -> Add/1
  Add/1 -> ConversiontoBits/1
  ConversiontoBits/1 -> Saturation/1
  In1/1 -> Bus Selector/1
  Data Type Conversion/1 -> rates/1
  Bus Selector/1 -> Bus Creator/1  "<phidot>"
  Bus Selector/2 -> Bus Creator/2  "<thetadot>"
  Bus Selector/3 -> Bus Creator/3  "<psidot>"
  Saturation/1 -> Data Type Conversion/1
  NoiseON/OFF/1 -> Add/2

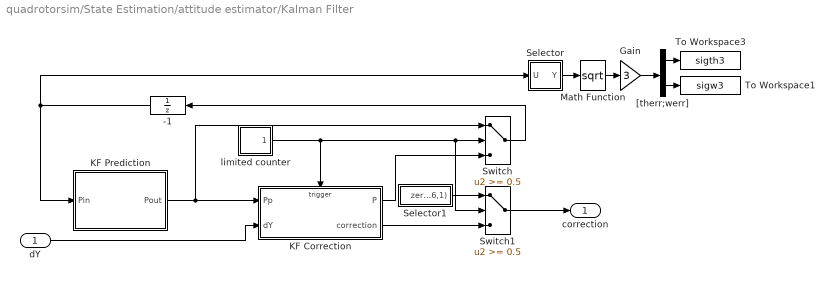
== system quadrotorsim/State Estimation/attitude estimator/Kalman Filter ==
  dY : Inport
  -1 : UnitDelay  SampleTime=-1
  Gain : Gain  Gain=3
  KF Correction : Subsystem
  KF Prediction : Subsystem
  Math Function : Math  Operator=sqrt  SaturateOnIntegerOverflow=on
  Selector : Subsystem
  Selector1 : Subsystem
  Switch : Switch  Threshold=0.5
  Switch1 : Switch  Threshold=0.5
  To Workspace1 : ToWorkspace  VariableName=sigw3  SampleTime=Tcapt
  To Workspace3 : ToWorkspace  VariableName=sigth3  SampleTime=Tcapt
  "[therr;werr]" : Demux  Outputs=[3 3]
  limited counter : Subsystem
  correction : Outport
  wires:
  Switch1/1 -> correction/1
  dY/1 -> KF Correction/2(dY)
  KF Correction/2(correction) -> Switch1/3
  Selector1/1(zeros(6,1)) -> Switch1/1
  Switch/1 -> -1/1
  limited counter/1(count) -> Switch1/2, Switch/2, KF Correction/Trigger
  KF Correction/1(P) -> Switch/3
  KF Prediction/1(Pout) -> Switch/1, KF Correction/1(Pp)
  -1/1 -> Selector/1(U), KF Prediction/1(Pin)
  "[therr;werr]"/2 -> To Workspace1/1
  "[therr;werr]"/1 -> To Workspace3/1
  Gain/1 -> "[therr;werr]"/1
  Math Function/1 -> Gain/1
  Selector/1(Y) -> Math Function/1

== system quadrotorsim/State Estimation/attitude estimator/angle metering ==
  i : Inport
  Saturation2 : Saturate  UpperLimit=delta_th_lim  LowerLimit=-delta_th_lim
  Sum2 : Sum  Inputs=|++  SaturateOnIntegerOverflow=on  InputSameDT=on  OutDataTypeStr=Inherit: Same as first input
  Sum5 : Sum  Inputs=+-|  SaturateOnIntegerOverflow=on  InputSameDT=on  OutDataTypeStr=Inherit: Same as first input
  Unit Delay7 : UnitDelay  InitialCondition=[0;0;0]  SampleTime=Tqint
  o : Outport
  wires:
  Saturation2/1 -> o/1, Sum5/2
  Sum2/1 -> Saturation2/1, Sum5/1
  Sum5/1 -> Unit Delay7/1
  Unit Delay7/1 -> Sum2/2
  i/1 -> Sum2/1

== system quadrotorsim/State Estimation/attitude estimator/bias metering ==
  i : Inport
  Saturation2 : Saturate  UpperLimit=delta_w_lim  LowerLimit=-delta_w_lim
  Sum2 : Sum  Inputs=|++  SaturateOnIntegerOverflow=on  InputSameDT=on  OutDataTypeStr=Inherit: Same as first input
  Sum5 : Sum  Inputs=+-|  SaturateOnIntegerOverflow=on  InputSameDT=on  OutDataTypeStr=Inherit: Same as first input
  Unit Delay7 : UnitDelay  InitialCondition=[0;0;0]  SampleTime=Tqint
  o : Outport
  wires:
  i/1 -> Sum2/1
  Unit Delay7/1 -> Sum2/2
  Sum5/1 -> Unit Delay7/1
  Sum2/1 -> Sum5/1, Saturation2/1
  Saturation2/1 -> Sum5/2, o/1

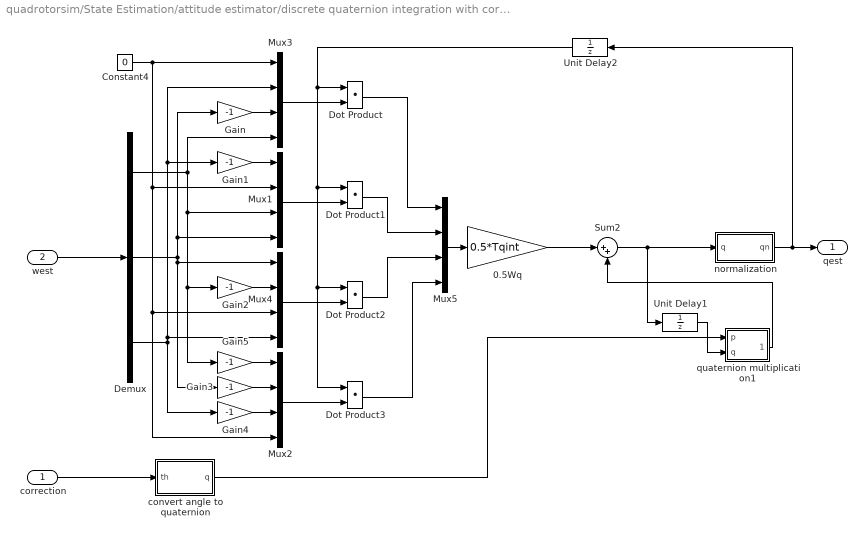
== system quadrotorsim/State Estimation/attitude estimator/discrete quaternion integration with correction ==
  correction : Inport
  west : Inport  Port=2
  0.5Wq : Gain  Gain=0.5*Tqint
  Constant4 : Constant  Value=0
  Demux : Demux  Outputs=3
  Dot Product{,1..3} (4 alike) : DotProduct  InputSameDT=on  OutDataTypeStr=Inherit: Inherit via internal rule
  Gain{,1..5} (6 alike) : Gain  Gain=-1
  Mux{1..5} (5 alike) : Mux
  Sum2 : Sum  Inputs=|++  SaturateOnIntegerOverflow=on  InputSameDT=on  OutDataTypeStr=Inherit: Same as first input
  Unit Delay1 : UnitDelay  InitialCondition=qest0  SampleTime=Tqint
  Unit Delay2 : UnitDelay  InitialCondition=qest0  SampleTime=Tqint
  convert angle to quaternion : Subsystem
  normalization : Subsystem
  quaternion multiplication1 : Subsystem
  qest : Outport
  wires:
  normalization/1(qn) -> qest/1, Unit Delay2/1
  0.5Wq/1 -> Sum2/1
  Mux5/1 -> 0.5Wq/1
  Dot Product3/1 -> Mux5/4
  Dot Product2/1 -> Mux5/3
  Dot Product1/1 -> Mux5/2
  Dot Product/1 -> Mux5/1
  Mux2/1 -> Dot Product3/2
  Mux4/1 -> Dot Product2/2
  Mux1/1 -> Dot Product1/2
  Mux3/1 -> Dot Product/2
  west/1 -> Demux/1
  Demux/3 -> Mux4/4, Mux3/2, Gain1/1, Gain4/1
  Demux/2 -> Mux4/1, Gain3/1, Mux1/4, Gain/1
  Demux/1 -> Gain2/1, Gain5/1, Mux1/3, Mux3/4
  Gain4/1 -> Mux2/3
  Gain3/1 -> Mux2/2
  Gain5/1 -> Mux2/1
  Gain1/1 -> Mux1/1
  Constant4/1 -> Mux4/3, Mux2/4, Mux1/2, Mux3/1
  Gain/1 -> Mux3/3
  Gain2/1 -> Mux4/2
  Sum2/1 -> normalization/1(q), Unit Delay1/1
  Unit Delay2/1 -> Dot Product/1, Dot Product1/1, Dot Product2/1, Dot Product3/1
  correction/1 -> convert angle to quaternion/1(th)
  convert angle to quaternion/1(q) -> quaternion multiplication1/1(p)
  quaternion multiplication1/1(p(x)q) -> Sum2/2
  Unit Delay1/1 -> quaternion multiplication1/2(q)

== system quadrotorsim/State Estimation/attitude estimator/quaternion inversion ==
  q : Inport
  Demux : Demux  Outputs=[3 1]
  Gain : Gain  Gain=-1
  Mux6 : Mux  Inputs=[3 1]
  invq : Outport
  wires:
  Demux/2 -> Mux6/2
  Gain/1 -> Mux6/1
  Demux/1 -> Gain/1
  Mux6/1 -> invq/1
  q/1 -> Demux/1

== system quadrotorsim/State Estimation/attitude estimator/quaternion multiplication ==
  p : Inport
  q : Inport  Port=2
  Demux : Demux  Outputs=[3 1]
  Demux1 : Demux  Outputs=[3 1]
  Dot Product4 : DotProduct  InputSameDT=on  OutDataTypeStr=Inherit: Inherit via internal rule
  Mux6 : Mux  Inputs=[3 1]
  Product : Product  SaturateOnIntegerOverflow=on  InputSameDT=on  OutDataTypeStr=Inherit: Same as first input
  Product1 : Product  SaturateOnIntegerOverflow=on  InputSameDT=on  OutDataTypeStr=Inherit: Same as first input
  Product2 : Product  SaturateOnIntegerOverflow=on  InputSameDT=on  OutDataTypeStr=Inherit: Same as first input
  Sum1 : Sum  Inputs=+-+  SaturateOnIntegerOverflow=on  InputSameDT=on  OutDataTypeStr=Inherit: Same as first input
  Sum2 : Sum  Inputs=-+|  SaturateOnIntegerOverflow=on  InputSameDT=on  OutDataTypeStr=Inherit: Same as first input
  cross1 : Subsystem
  p(x)q : Outport
  wires:
  Mux6/1 -> p(x)q/1
  Sum2/1 -> Mux6/2
  Dot Product4/1 -> Sum2/1
  Sum1/1 -> Mux6/1
  Product1/1 -> Sum1/3
  cross1/1(axb) -> Sum1/2
  Product/1 -> Sum1/1
  Demux1/1 -> Dot Product4/1, cross1/2(b), Product1/2
  Demux/2 -> Product1/1, Product2/1
  Demux1/2 -> Product/2, Product2/2
  Demux/1 -> Dot Product4/2, cross1/1(a), Product/1
  q/1 -> Demux1/1
  p/1 -> Demux/1
  Product2/1 -> Sum2/2

== system quadrotorsim/State Estimation/kinematics: dq/dt = 1/2 Wq/normalization ==
  q : Inport
  Dot Product : DotProduct  InputSameDT=on  OutDataTypeStr=Inherit: Inherit via internal rule
  Math Function : Math  Operator=sqrt  SaturateOnIntegerOverflow=on
  Math Function1 : Math  Operator=reciprocal  SaturateOnIntegerOverflow=on
  Product : Product  SaturateOnIntegerOverflow=on  InputSameDT=on  OutDataTypeStr=Inherit: Same as first input
  qn : Outport
  wires:
  q/1 -> Dot Product/1, Dot Product/2, Product/1
  Dot Product/1 -> Math Function/1
  Math Function/1 -> Math Function1/1
  Math Function1/1 -> Product/2
  Product/1 -> qn/1

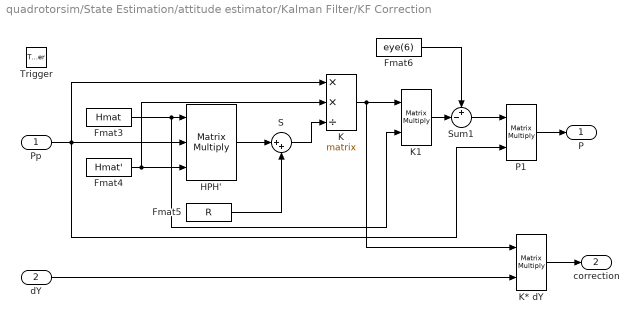
== system quadrotorsim/State Estimation/attitude estimator/Kalman Filter/KF Correction ==
  Pp : Inport
  dY : Inport  Port=2
  Trigger : TriggerPort  TriggerType=falling  VariantControl=(inherit)
  Fmat3 : Constant  Value=Hmat  VectorParams1D=off
  Fmat4 : Constant  Value=Hmat'  VectorParams1D=off
  Fmat5 : Constant  Value=R  VectorParams1D=off
  Fmat6 : Constant  Value=eye(6)  VectorParams1D=off
  HPH' : Product  Inputs=***  Multiplication=Matrix(*)  RndMeth=Zero
  K : Product  Inputs=**/  Multiplication=Matrix(*)  RndMeth=Zero
  K* dY : Product  Inputs=**  Multiplication=Matrix(*)  RndMeth=Zero
  K1 : Product  Inputs=**  Multiplication=Matrix(*)  RndMeth=Zero
  P1 : Product  Inputs=**  Multiplication=Matrix(*)  RndMeth=Zero
  S : Sum  Inputs=|++  SaturateOnIntegerOverflow=on  InputSameDT=on  OutDataTypeStr=Inherit: Same as first input
  Sum1 : Sum  Inputs=+-|  SaturateOnIntegerOverflow=on  InputSameDT=on  OutDataTypeStr=Inherit: Same as first input
  P : Outport
  correction : Outport  Port=2
  wires:
  K* dY/1 -> correction/1
  dY/1 -> K* dY/2
  Fmat3/1 -> K1/2, HPH'/1
  Fmat4/1 -> K/2, HPH'/3
  HPH'/1 -> S/1
  Fmat5/1 -> S/2
  Pp/1 -> HPH'/2, P1/2, K/1
  S/1 -> K/3
  K/1 -> K* dY/1, K1/1
  Fmat6/1 -> Sum1/1
  K1/1 -> Sum1/2
  Sum1/1 -> P1/1
  P1/1 -> P/1

== system quadrotorsim/State Estimation/attitude estimator/Kalman Filter/KF Prediction ==
  note: The state propagation (x=Ax+Bu) is done in the simulation integration portion
  Pin : Inport
  FPF' : Product  Inputs=***  Multiplication=Matrix(*)  RndMeth=Zero
  Fmat : Constant  Value=Fmat  VectorParams1D=off
  Fmat1 : Constant  Value=Fmat'  VectorParams1D=off
  Fmat2 : Constant  Value=Q  VectorParams1D=off
  Pp : Sum  Inputs=|++  SaturateOnIntegerOverflow=on  InputSameDT=on  OutDataTypeStr=Inherit: Same as first input
  Pout : Outport
  wires:
  Pp/1 -> Pout/1
  Pin/1 -> FPF'/2
  Fmat/1 -> FPF'/1
  Fmat1/1 -> FPF'/3
  FPF'/1 -> Pp/1
  Fmat2/1 -> Pp/2

== system quadrotorsim/State Estimation/attitude estimator/Kalman Filter/Selector ==
  U : Inport
  Mux2 : Mux  Inputs=6
  Selector1 : Selector  NumberOfDimensions=2  InputPortWidth=36  IndexOptions=Index vector (dialog),Index vector (dialog)  Indices=1,1  OutputSizes=1,1
  Selector2 : Selector  NumberOfDimensions=2  InputPortWidth=36  IndexOptions=Index vector (dialog),Index vector (dialog)  Indices=2,2  OutputSizes=1,1
  Selector3 : Selector  NumberOfDimensions=2  InputPortWidth=36  IndexOptions=Index vector (dialog),Index vector (dialog)  Indices=3,3  OutputSizes=1,1
  Selector4 : Selector  NumberOfDimensions=2  InputPortWidth=36  IndexOptions=Index vector (dialog),Index vector (dialog)  Indices=4,4  OutputSizes=1,1
  Selector5 : Selector  NumberOfDimensions=2  InputPortWidth=36  IndexOptions=Index vector (dialog),Index vector (dialog)  Indices=5,5  OutputSizes=1,1
  Selector6 : Selector  NumberOfDimensions=2  InputPortWidth=36  IndexOptions=Index vector (dialog),Index vector (dialog)  Indices=6,6  OutputSizes=1,1
  Y : Outport
  wires:
  Mux2/1 -> Y/1
  Selector6/1 -> Mux2/6
  Selector5/1 -> Mux2/5
  Selector4/1 -> Mux2/4
  Selector3/1 -> Mux2/3
  Selector2/1 -> Mux2/2
  Selector1/1 -> Mux2/1
  U/1 -> Selector6/1, Selector5/1, Selector4/1, Selector3/1, Selector2/1, Selector1/1

== system quadrotorsim/State Estimation/attitude estimator/Kalman Filter/Selector1 ==
  Fmat{1..6} (6 alike) : Constant  Value=0  VectorParams1D=off
  Mux2 : Mux  Inputs=6
  zeros(6,1) : Outport
  wires:
  Fmat1/1 -> Mux2/1
  Fmat3/1 -> Mux2/2
  Fmat2/1 -> Mux2/3
  Fmat4/1 -> Mux2/4
  Fmat6/1 -> Mux2/5
  Fmat5/1 -> Mux2/6
  Mux2/1 -> zeros(6,1)/1

== system quadrotorsim/State Estimation/attitude estimator/Kalman Filter/limited counter ==
  -1 : UnitDelay  InitialCondition=-1  SampleTime=TkfProp
  Fmat1 : Constant  Value=-1  VectorParams1D=off
  Fmat7 : Constant  VectorParams1D=off
  Pp : Sum  Inputs=|++  SaturateOnIntegerOverflow=on  InputSameDT=on  OutDataTypeStr=Inherit: Same as first input
  Switch : Switch  Threshold=KfupdatePeriodInCycle-1.5
  To Workspace3 : ToWorkspace  VariableName=count  SampleTime=Tcapt
  count : Outport
  wires:
  Pp/1 -> To Workspace3/1, count/1, Switch/3, Switch/2
  Fmat1/1 -> Switch/1
  -1/1 -> Pp/2
  Switch/1 -> -1/1
  Fmat7/1 -> Pp/1

== system quadrotorsim/State Estimation/attitude estimator/discrete quaternion integration with correction/convert angle to quaternion ==
  th : Inport
  Constant4 : Constant
  Dot Product : DotProduct  InputSameDT=on  OutDataTypeStr=Inherit: Inherit via internal rule
  Gain3 : Gain  Gain=0.5
  Math Function : Math  Operator=sqrt  SaturateOnIntegerOverflow=on
  Mux3 : Mux  Inputs=[3 1]
  Sum1 : Sum  Inputs=|-+  SaturateOnIntegerOverflow=on  InputSameDT=on  OutDataTypeStr=Inherit: Same as first input
  q : Outport
  wires:
  Gain3/1 -> Mux3/1, Dot Product/2, Dot Product/1
  Mux3/1 -> q/1
  Math Function/1 -> Mux3/2
  Sum1/1 -> Math Function/1
  Constant4/1 -> Sum1/2
  Dot Product/1 -> Sum1/1
  th/1 -> Gain3/1

== system quadrotorsim/State Estimation/attitude estimator/discrete quaternion integration with correction/normalization ==
  q : Inport
  Dot Product : DotProduct  InputSameDT=on  OutDataTypeStr=Inherit: Inherit via internal rule
  Math Function : Math  Operator=sqrt  SaturateOnIntegerOverflow=on
  Math Function1 : Math  Operator=reciprocal  SaturateOnIntegerOverflow=on
  Product : Product  SaturateOnIntegerOverflow=on  InputSameDT=on  OutDataTypeStr=Inherit: Same as first input
  qn : Outport
  wires:
  Product/1 -> qn/1
  Math Function1/1 -> Product/2
  Math Function/1 -> Math Function1/1
  Dot Product/1 -> Math Function/1
  q/1 -> Product/1, Dot Product/2, Dot Product/1

== system quadrotorsim/State Estimation/attitude estimator/discrete quaternion integration with correction/quaternion multiplication1 ==
  p : Inport
  q : Inport  Port=2
  Demux : Demux  Outputs=[3 1]
  Demux1 : Demux  Outputs=[3 1]
  Dot Product4 : DotProduct  InputSameDT=on  OutDataTypeStr=Inherit: Inherit via internal rule
  Mux6 : Mux  Inputs=[3 1]
  Product : Product  SaturateOnIntegerOverflow=on  InputSameDT=on  OutDataTypeStr=Inherit: Same as first input
  Product1 : Product  SaturateOnIntegerOverflow=on  InputSameDT=on  OutDataTypeStr=Inherit: Same as first input
  Product2 : Product  SaturateOnIntegerOverflow=on  InputSameDT=on  OutDataTypeStr=Inherit: Same as first input
  Sum1 : Sum  Inputs=+-+  SaturateOnIntegerOverflow=on  InputSameDT=on  OutDataTypeStr=Inherit: Same as first input
  Sum2 : Sum  Inputs=-+|  SaturateOnIntegerOverflow=on  InputSameDT=on  OutDataTypeStr=Inherit: Same as first input
  cross1 : Subsystem
  p(x)q : Outport
  wires:
  Product2/1 -> Sum2/2
  p/1 -> Demux/1
  q/1 -> Demux1/1
  Demux/1 -> Product/1, cross1/1(a), Dot Product4/2
  Demux1/2 -> Product2/2, Product/2
  Demux/2 -> Product2/1, Product1/1
  Demux1/1 -> Product1/2, cross1/2(b), Dot Product4/1
  Product/1 -> Sum1/1
  cross1/1(axb) -> Sum1/2
  Product1/1 -> Sum1/3
  Sum1/1 -> Mux6/1
  Dot Product4/1 -> Sum2/1
  Sum2/1 -> Mux6/2
  Mux6/1 -> p(x)q/1

== system quadrotorsim/State Estimation/attitude estimator/quaternion multiplication/cross1 ==
  a : Inport
  b : Inport  Port=2
  Demux : Demux  Outputs=3
  Demux1 : Demux  Outputs=3
  Mux : Mux  Inputs=3
  Product{,1..5} (6 alike) : Product  SaturateOnIntegerOverflow=on  InputSameDT=on  OutDataTypeStr=Inherit: Same as first input
  Sum : Sum  Inputs=|+-  SaturateOnIntegerOverflow=on  InputSameDT=on  OutDataTypeStr=Inherit: Same as first input
  Sum1 : Sum  Inputs=|+-  SaturateOnIntegerOverflow=on  InputSameDT=on  OutDataTypeStr=Inherit: Same as first input
  Sum2 : Sum  Inputs=|+-  SaturateOnIntegerOverflow=on  InputSameDT=on  OutDataTypeStr=Inherit: Same as first input
  axb : Outport
  wires:
  Sum2/1 -> Mux/3
  Product5/1 -> Sum2/2
  Product4/1 -> Sum2/1
  Demux1/1 -> Product5/2, Product2/2
  Demux/2 -> Product5/1, Product/1
  Demux/1 -> Product4/1, Product3/1
  Demux1/2 -> Product4/2, Product1/2
  Sum1/1 -> Mux/2
  Product3/1 -> Sum1/2
  Product2/1 -> Sum1/1
  Demux1/3 -> Product3/2, Product/2
  Demux/3 -> Product2/1, Product1/1
  Mux/1 -> axb/1
  Sum/1 -> Mux/1
  Product1/1 -> Sum/2
  Product/1 -> Sum/1
  b/1 -> Demux1/1
  a/1 -> Demux/1

== system quadrotorsim/State Estimation/attitude estimator/discrete quaternion integration with correction/quaternion multiplication1/cross1 ==
  a : Inport
  b : Inport  Port=2
  Demux : Demux  Outputs=3
  Demux1 : Demux  Outputs=3
  Mux : Mux  Inputs=3
  Product{,1..5} (6 alike) : Product  SaturateOnIntegerOverflow=on  InputSameDT=on  OutDataTypeStr=Inherit: Same as first input
  Sum : Sum  Inputs=|+-  SaturateOnIntegerOverflow=on  InputSameDT=on  OutDataTypeStr=Inherit: Same as first input
  Sum1 : Sum  Inputs=|+-  SaturateOnIntegerOverflow=on  InputSameDT=on  OutDataTypeStr=Inherit: Same as first input
  Sum2 : Sum  Inputs=|+-  SaturateOnIntegerOverflow=on  InputSameDT=on  OutDataTypeStr=Inherit: Same as first input
  axb : Outport
  wires:
  a/1 -> Demux/1
  b/1 -> Demux1/1
  Product/1 -> Sum/1
  Product1/1 -> Sum/2
  Sum/1 -> Mux/1
  Mux/1 -> axb/1
  Demux/3 -> Product1/1, Product2/1
  Demux1/3 -> Product/2, Product3/2
  Product2/1 -> Sum1/1
  Product3/1 -> Sum1/2
  Sum1/1 -> Mux/2
  Demux1/2 -> Product1/2, Product4/2
  Demux/1 -> Product3/1, Product4/1
  Demux/2 -> Product/1, Product5/1
  Demux1/1 -> Product2/2, Product5/2
  Product4/1 -> Sum2/1
  Product5/1 -> Sum2/2
  Sum2/1 -> Mux/3
